simulink library "PALANCA"  (R2025b)
settings: Solver=VariableStepAuto  StartTime=0.0  StopTime=10.0  RelTol=1e-3
settings Model: Creator=joshu  LastModifiedBy=joshu

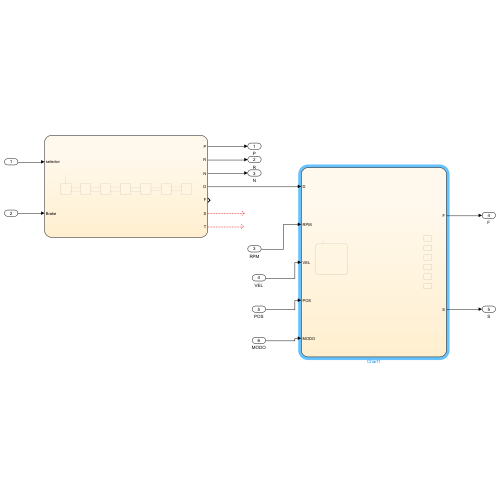
[thumbnail: Simulink's stored preview of the top-level diagram]
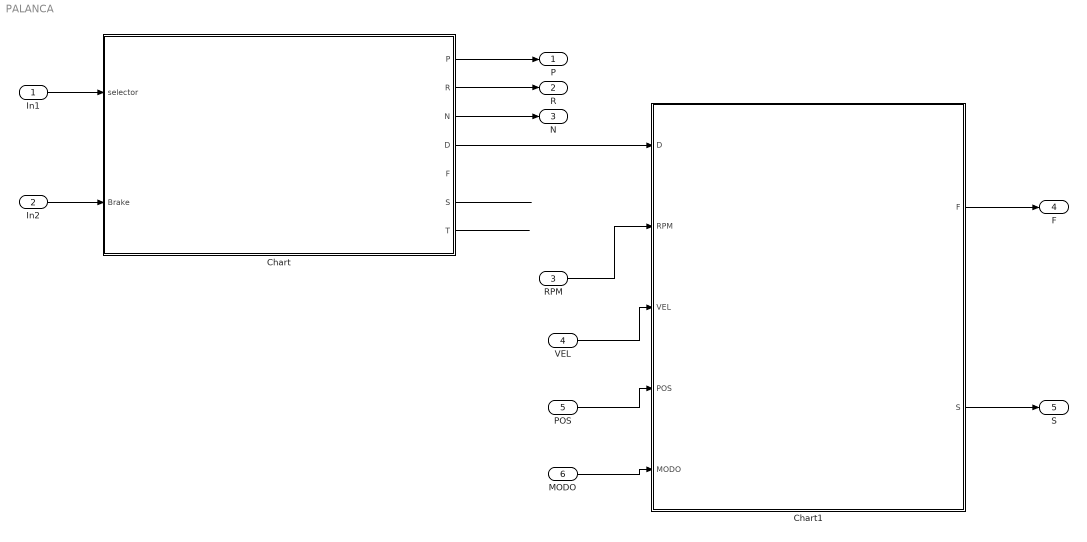
== system PALANCA ==
  In1 : Inport
  In2 : Inport  Port=2
  RPM : Inport  Port=3
  VEL : Inport  Port=4
  POS : Inport  Port=5
  MODO : Inport  Port=6
  Chart : Stateflow chart  TreatAsAtomicUnit=on
      settings: PortSchema="{\"entries\":[{\"content\":{\"sides\":[{\"content\":{\"connectorIds\":[\"In1\",\"In2\"]},\"type\":\"ConnectorPlacement.EquallySpacedRectSide\",\"uuid\":\"e4c66ebb-7da8-44e5-99b8-7444c5aa35cd\"},{\"content\":{\"connectorIds\":[\"Out4\",\"Out5\",\"Out3\",\"Out2\",\"Out1\",\"Out6\",\"Out7\"],\"side\":\"RIGHT\"},\"type\":\"ConnectorPlacement.EquallySpacedRectSide\",\"uuid\":\"c40422dc-742f-4821-91a3-3b1c75b25b89\"},{\"content\":{\"side\":\"TOP\"},\"type\":\"ConnectorPlacement.EquallySpacedRectSide\",\"uuid\":\"68be5695-d827-488a-8b92-864f7f5dd84f\"}]},\"type\":\"ConnectorPlacement.EquallySpacedConnector\",\"uuid\":\"fee762eb-152d-4b84-a6dc-7bcd9436287d\"}],\"packageUris\":[\"http://schema.mathworks.com/mf0/Connector/R2020b\"],\"version\":\"1.0\"}"
  Chart1 : Stateflow chart  TreatAsAtomicUnit=on
  P : Outport  OutDataTypeStr=uint8
  R : Outport  Port=2  OutDataTypeStr=uint8
  N : Outport  Port=3  OutDataTypeStr=uint8
  F : Outport  Port=4
  S : Outport  Port=5
  wires:
  Chart/3(N) -> N/1
  In1/1 -> Chart/1(selector)
  In2/1 -> Chart/2(Brake)
  Chart/4(P) -> P/1
  Chart/5(R) -> R/1
  Chart/6(S) -> ?
  Chart/2(D) -> Chart1/1(D)
  Chart/7(T) -> ?
  RPM/1 -> Chart1/2(RPM)
  VEL/1 -> Chart1/3(VEL)
  POS/1 -> Chart1/4(POS)
  MODO/1 -> Chart1/5(MODO)
  Chart1/1(F) -> F/1
  Chart1/2(S) -> S/1

== stateflow chart PALANCA/Chart1 ==
  state PRIMERA
  state DRIVE
  state SEGUNDA
  state TERCERA
  state CUARTA
  state QUINTA
  state SEXTA
  (default) -> DRIVE
  data: D input; RPM input; VEL input; POS input; MODO input; F output; S output

== stateflow chart PALANCA/Chart ==
  state parking
    during:
    P=1;
    R=0;
    N=0;
    D=0;
    F=0;
    S=0;
    T=0;
  state reverse
    during:
    P=0;
    R=1;
    N=0;
    D=0;
    F=0;
    S=0;
    T=0;
  state neutral
    during:
    P=0;
    R=0;
    N=1;
    D=0;
    F=0;
    S=0;
    T=0;
  state drive
    during:
    P=0;
    R=0;
    N=0;
    D=1;
    F=0;
    S=0;
    T=0;
  state primera
    during:
    P=0;
    R=0;
    N=0;
    D=0;
    F=1;
    S=0;
    T=0;
  state segunda
    during:
    P=0;
    R=0;
    N=0;
    D=0;
    F=0;
    S=1;
    T=0;
  state tercera
    during:
    P=0;
    R=0;
    N=0;
    D=0;
    F=0;
    S=0;
    T=1;
  (default) -> parking
  neutral -> drive [order 1] : [selector==4]
  segunda -> tercera [order 1] : [selector==32]
  reverse -> neutral [order 1] : [selector==2]
  primera -> segunda [order 1] : [selector==16]
  parking -> reverse : [selector==1 && Brake == 1]
  drive -> primera [order 1] : [selector==8]
  segunda -> primera [order 2] : [selector==8]
  tercera -> segunda : [selector==16]
  primera -> drive [order 2] : [selector==4]
  neutral -> reverse [order 2] : [selector==1]
  reverse -> parking [order 2] : [selector==0 && Brake == 1]
  drive -> neutral [order 2] : [selector==2]
  data: selector input uint8; F output uint8; D output uint8; N output uint8; P output uint8; R output uint8; S output uint8; T output uint8; Brake input uint8
